simulink library "SEMACE4_IN"  (R2021b)
settings: Solver=VariableStepAuto  StartTime=0.0  StopTime=10.0  RelTol=1e-3
values from neighbouring files (symbols this model uses):
  dataSEMACE = 60.0    [applicationDD.sldd]    (also in dataSEMACE.mat = ; dataSEMACE_DD.sldd)
settings Model: Creator=ACH  LastModifiedBy=C83127

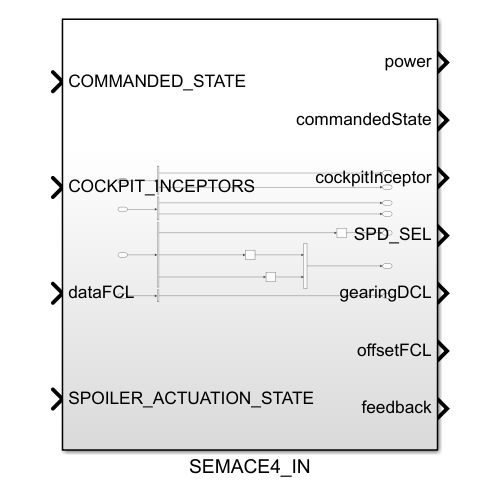
[thumbnail: Simulink's stored preview of the top-level diagram]
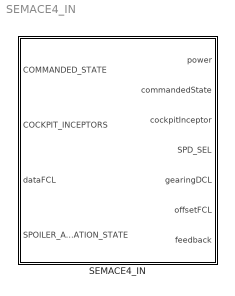
== system SEMACE4_IN ==
  SEMACE4_IN : Subsystem

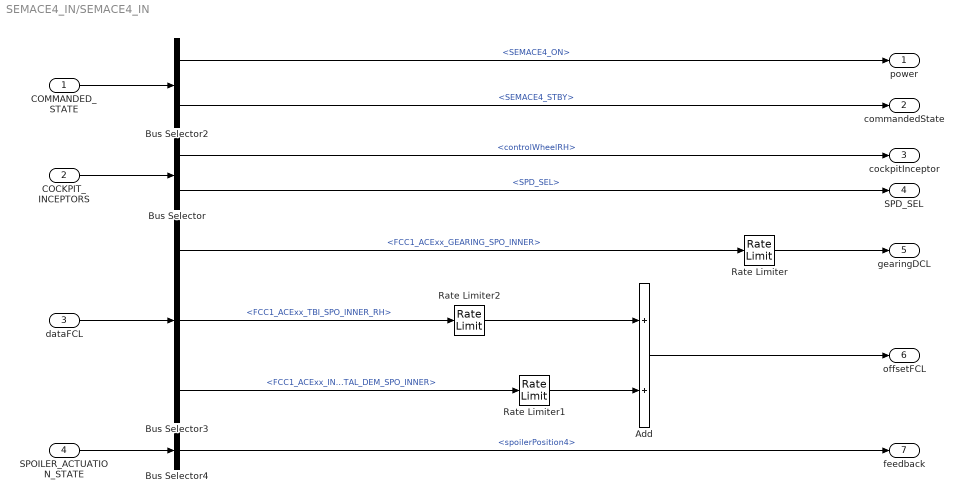
== system SEMACE4_IN/SEMACE4_IN ==
  COMMANDED_STATE : Inport  OutDataTypeStr=Bus: COMMANDED_STATE
  COCKPIT_INCEPTORS : Inport  Port=2  OutDataTypeStr=Bus: COCKPIT_INCEPTORS
  dataFCL : Inport  Port=3  OutDataTypeStr=Bus: FCC1_TC_TX_12_SPOILER_INNER
  SPOILER_ACTUATION_STATE : Inport  Port=4  OutDataTypeStr=Bus: SPOILER_ACTUATION_STATE
  Add : Sum
  Bus Selector : BusSelector  OutputSignals=controlWheelRH,SPD_SEL
  Bus Selector2 : BusSelector  OutputSignals=SEMACE4_ON,SEMACE4_STBY
  Bus Selector3 : BusSelector  OutputSignals=FCC1_ACExx_GEARING_SPO_INNER,FCC1_ACExx_TBI_SPO_INNER_RH,FCC1_ACExx_INCREMENTAL_DEM_SPO_INNER
  Bus Selector4 : BusSelector  OutputSignals=spoilerPosition4
  Rate Limiter : RateLimiter  RisingSlewLimit=dataSEMACE.rateLimiterGearing  FallingSlewLimit=-dataSEMACE.rateLimiterGearing  SampleTimeMode=inherited
      settings: AttributesFormatString=|
      | %<RisingSlewLimit>
      | %<FallingSlewLimit>
  Rate Limiter1 : RateLimiter  RisingSlewLimit=dataSEMACE.rateLimiterSymmetric  FallingSlewLimit=-dataSEMACE.rateLimiterSymmetric  SampleTimeMode=inherited
      settings: AttributesFormatString=|
      | %<RisingSlewLimit>
      | %<FallingSlewLimit>
  Rate Limiter2 : RateLimiter  RisingSlewLimit=dataSEMACE.rateLimiterTBI  FallingSlewLimit=-dataSEMACE.rateLimiterTBI  SampleTimeMode=inherited
      settings: AttributesFormatString=|
      | %<RisingSlewLimit>
      | %<FallingSlewLimit>
  power : Outport
  commandedState : Outport  Port=2
  cockpitInceptor : Outport  Port=3
  SPD_SEL : Outport  Port=4
  gearingDCL : Outport  Port=5
  offsetFCL : Outport  Port=6
  feedback : Outport  Port=7
  wires:
  Bus Selector3/2 -> Rate Limiter2/1  "<FCC1_ACExx_TBI_SPO_INNER_RH>"
  Add/1 -> offsetFCL/1
  Bus Selector3/3 -> Rate Limiter1/1  "<FCC1_ACExx_INCREMENTAL_DEM_SPO_INNER>"
  SPOILER_ACTUATION_STATE/1 -> Bus Selector4/1
  Bus Selector2/1 -> power/1  "<SEMACE4_ON>"
  Bus Selector4/1 -> feedback/1  "<spoilerPosition4>"
  COMMANDED_STATE/1 -> Bus Selector2/1
  dataFCL/1 -> Bus Selector3/1
  COCKPIT_INCEPTORS/1 -> Bus Selector/1
  Bus Selector/1 -> cockpitInceptor/1  "<controlWheelRH>"
  Bus Selector3/1 -> Rate Limiter/1  "<FCC1_ACExx_GEARING_SPO_INNER>"
  Rate Limiter1/1 -> Add/2
  Rate Limiter/1 -> gearingDCL/1
  Rate Limiter2/1 -> Add/1
  Bus Selector2/2 -> commandedState/1  "<SEMACE4_STBY>"
  Bus Selector/2 -> SPD_SEL/1  "<SPD_SEL>"
